simulink model "data_generator_sim"  (R2021a)
settings: Solver=VariableStepAuto  StartTime=0.0  StopTime=6  RelTol=1e-3
values from neighbouring files (symbols this model uses):
  A = [ ... (first row only)    [data_generator.m]
  B = [ ... (first row only)    [data_generator.m]
  C = eye(6,6)    [data_generator.m]
  D = zeros(6,2)    [data_generator.m]
  x0 = pi*[1, 1, -1.5, 1, -1, 1]    [data_generator.m]
libraries: mpclib x2
settings Model: PacingRate=0.450000  Creator=alexmeyer  LastModifiedBy=alexmeyer

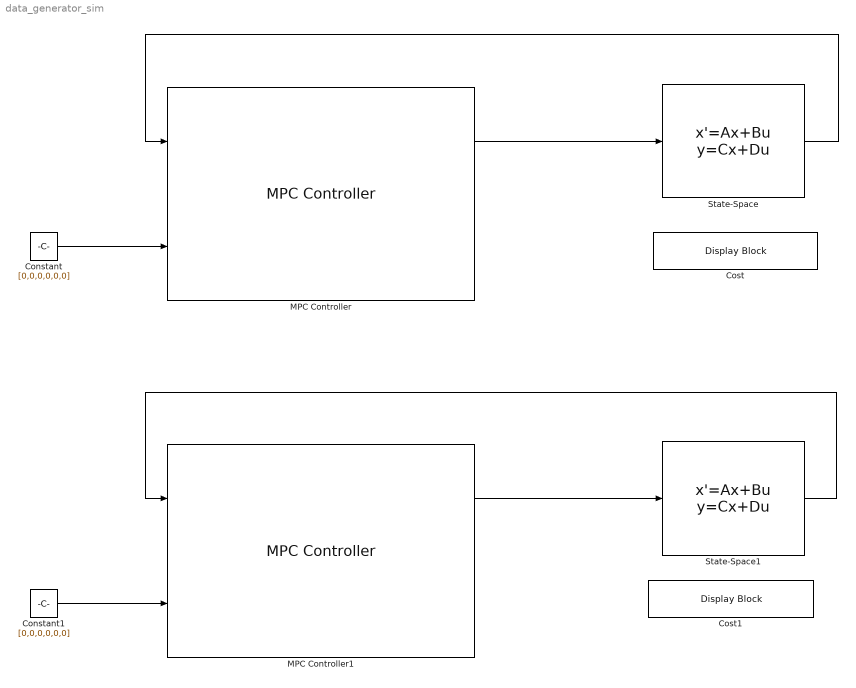
== system data_generator_sim ==
  Constant : Constant  Value=[0,0,0,0,0,0]
  Constant1 : Constant  Value=[0,0,0,0,0,0]
  Cost : DisplayBlock  LabelPosition=Hide  Format=shortEng  Transparency=1
  Cost1 : DisplayBlock  LabelPosition=Hide  Format=shortEng  Transparency=1
  MPC Controller : mpclib/MPC Controller  SCDEnableBlockLinearizationSpecification=on  mpcobj=controller_ipopt  is_multiple=0  enable_value=0  return_u0=off  updateMPCinCallerWorkspace=on  md_inport=off  mv_inport=off  uref_inport=off  return_cost=on  return_mvseq=off  return_qpstatus=off  return_xseq=off  return_state=off  return_ovseq=off  state_inport=off  umin_inport=off  umax_inport=off  ymin_inport=off  ymax_inport=off  cc_inport=off  ywt_inport=off  uwt_inport=off  duwt_inport=off  rhoeps_inport=off  pm_inport=off  MaximumP=20  HorizonChoice=FixedHorizon  n_ts=0.1  n_p=20  n_mv=2  n_md=0  n_ud=0  n_mo=6  n_uo=0  BlockDataType=double  SampleTimeInherited=off  switch_inport=off
  MPC Controller1 : mpclib/MPC Controller  SCDEnableBlockLinearizationSpecification=on  mpcobj=controller_other  is_multiple=0  enable_value=0  return_u0=off  updateMPCinCallerWorkspace=on  md_inport=off  mv_inport=off  uref_inport=off  return_cost=on  return_mvseq=off  return_qpstatus=off  return_xseq=off  return_state=off  return_ovseq=off  state_inport=off  umin_inport=off  umax_inport=off  ymin_inport=off  ymax_inport=off  cc_inport=off  ywt_inport=off  uwt_inport=off  duwt_inport=off  rhoeps_inport=off  pm_inport=off  MaximumP=20  HorizonChoice=FixedHorizon  n_ts=0.1  n_p=20  n_mv=2  n_md=0  n_ud=0  n_mo=6  n_uo=0  BlockDataType=double  SampleTimeInherited=off  switch_inport=off
  State-Space : StateSpace  A=A  B=B  C=C  D=D  InitialCondition=x0
  State-Space1 : StateSpace  A=A  B=B  C=C  D=D  InitialCondition=x0
  wires:
  MPC Controller/1 -> State-Space/1
  Constant/1 -> MPC Controller/2
  State-Space/1 -> MPC Controller/1
  State-Space1/1 -> MPC Controller1/1
  Constant1/1 -> MPC Controller1/2
  MPC Controller1/1 -> State-Space1/1
